simulink library "hgFilter"  (R2016b)
settings: Solver=VariableStepAuto  StartTime=0.0  StopTime=10.0  RelTol=1e-3
libraries: hgFilter x3
settings Model: Creator=Norris  LastModifiedBy=Norris

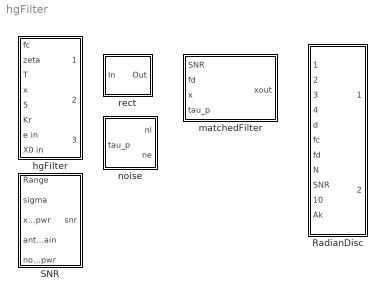
== system hgFilter ==
  RadianDisc : Subsystem
  SNR : Subsystem  Description=Calculates the SNR given several inputs, including range and RCS (sigma)
  hgFilter : Subsystem
  matchedFilter : Subsystem
  noise : Subsystem  Description=|
      | Takes in Tau_p and T (time step) and outputs all three noise coeffs. Note that currently Ak must be set 
      | in the workspace as 'Ak' for this block to function. Additionally, this version does not account for
      | multiple targets (there is only one Ak)
  rect : Subsystem  Description=Returns 1 if the mag of IN is 0.5 or less. Returns 0 otherwise

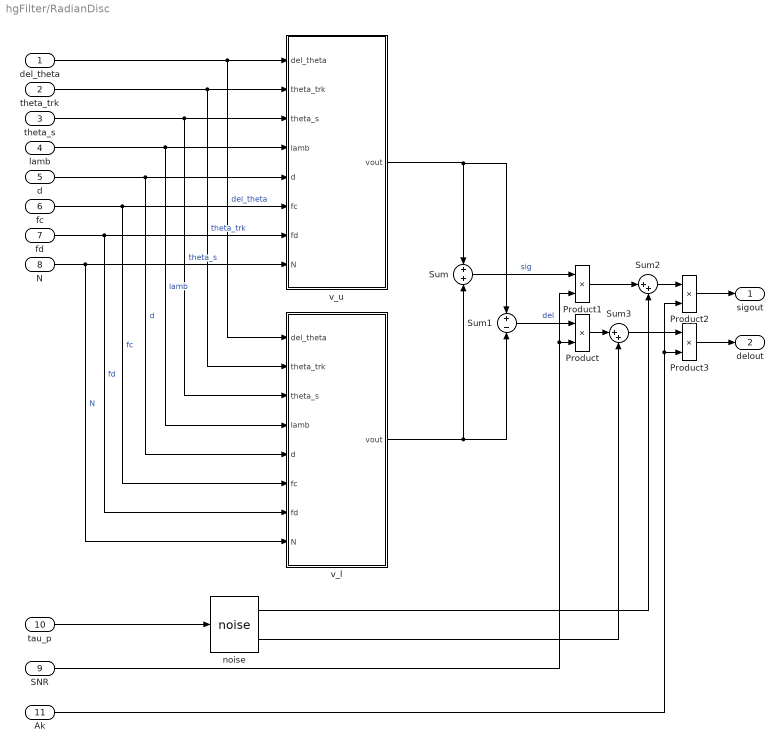
== system hgFilter/RadianDisc ==
  del_theta : Inport
  theta_trk : Inport  Port=2
  theta_s : Inport  Port=3
  lamb : Inport  Port=4
  d : Inport  Port=5
  fc : Inport  Port=6
  fd : Inport  Port=7
  N : Inport  Port=8
  SNR : Inport  Port=9
  tau_p : Inport  Port=10
  Ak : Inport  Port=11
  Product{,1..3} (4 alike) : Product
  Sum : Sum
  Sum1 : Sum  Inputs=+-
  Sum2 : Sum  Inputs=|++
  Sum3 : Sum  Inputs=|++
  noise : hgFilter/noise  Description=|
      | Takes in Tau_p and T (time step) and outputs all three noise coeffs. Note that currently Ak must be set 
      | in the workspace as 'Ak' for this block to function. Additionally, this version does not account for
      | multiple targets (there is only one Ak)
  v_l : Subsystem
  v_u : Subsystem
  sigout : Outport
  delout : Outport  Port=2
  wires:
  tau_p/1 -> noise/1
  Product2/1 -> sigout/1
  Sum3/1 -> Product3/1
  Sum2/1 -> Product2/1
  Product/1 -> Sum3/1
  Product1/1 -> Sum2/1
  del_theta/1 -> v_l/1(del_theta), v_u/1(del_theta)  "del_theta"
  theta_trk/1 -> v_l/2(theta_trk), v_u/2(theta_trk)  "theta_trk"
  theta_s/1 -> v_l/3(theta_s), v_u/3(theta_s)  "theta_s"
  lamb/1 -> v_l/4(lamb), v_u/4(lamb)  "lamb"
  d/1 -> v_l/5(d), v_u/5(d)  "d"
  fc/1 -> v_l/6(fc), v_u/6(fc)  "fc"
  fd/1 -> v_l/7(fd), v_u/7(fd)  "fd"
  N/1 -> v_l/8(N), v_u/8(N)  "N"
  v_l/1(vout) -> Sum1/2, Sum/2
  v_u/1(vout) -> Sum1/1, Sum/1
  Sum/1 -> Product1/1  "sig"
  Sum1/1 -> Product/1  "del"
  SNR/1 -> Product1/2, Product/2
  Product3/1 -> delout/1
  noise/1 -> Sum2/2
  noise/2 -> Sum3/2
  Ak/1 -> Product2/2, Product3/2

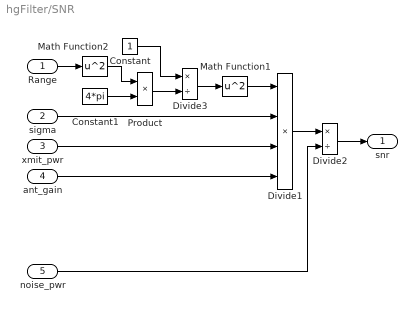
== system hgFilter/SNR ==
  Range : Inport
  sigma : Inport  Port=2
  xmit_pwr : Inport  Port=3
  ant_gain : Inport  Port=4
  noise_pwr : Inport  Port=5
  Constant : Constant
  Constant1 : Constant  Value=4*pi
  Divide1 : Product  Inputs=****
  Divide2 : Product  Inputs=*/
  Divide3 : Product  Inputs=*/
  Math Function1 : Math  Operator=square  SaturateOnIntegerOverflow=on
  Math Function2 : Math  Operator=square  SaturateOnIntegerOverflow=on
  Product : Product
  snr : Outport
  wires:
  Divide2/1 -> snr/1
  noise_pwr/1 -> Divide2/2
  xmit_pwr/1 -> Divide1/3
  sigma/1 -> Divide1/2
  ant_gain/1 -> Divide1/4
  Divide3/1 -> Math Function1/1
  Math Function1/1 -> Divide1/1
  Constant/1 -> Divide3/1
  Product/1 -> Divide3/2
  Range/1 -> Math Function2/1
  Constant1/1 -> Product/2
  Divide1/1 -> Divide2/1
  Math Function2/1 -> Product/1

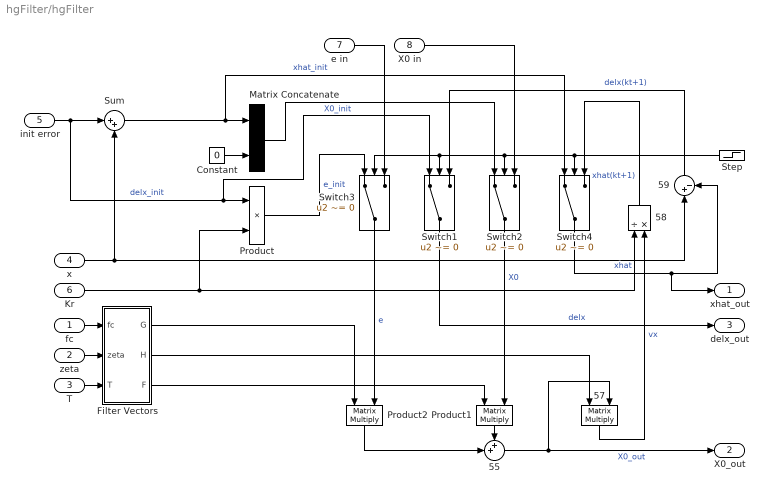
== system hgFilter/hgFilter ==
  fc : Inport
  zeta : Inport  Port=2
  T : Inport  Port=3
  x : Inport  Port=4
  init error : Inport  Port=5
  Kr : Inport  Port=6
  e in : Inport  Port=7
  X0 in : Inport  Port=8
  55 : Sum  Inputs=++|
  57 : Product  Multiplication=Matrix(*)
  58 : Product  Inputs=/*
  59 : Sum  Inputs=|+-
  Constant : Constant  Value=0
  Filter Vectors : Subsystem  TreatAsAtomicUnit=on
  Matrix Concatenate : Concatenate  Mode=Multidimensional array
  Product : Product
  Product1 : Product  Multiplication=Matrix(*)
  Product2 : Product  Multiplication=Matrix(*)
  Step : Step  Time=0.01  Before=1  After=0  SampleTime=0
  Sum : Sum  Inputs=|++
  Switch{1..4} (4 alike) : Switch  Criteria=u2 ~= 0  Threshold=0.5
  xhat_out : Outport
  X0_out : Outport  Port=2
  delx_out : Outport  Port=3
  wires:
  X0 in/1 -> Switch2/3
  59/1 -> Switch1/3  "delx(kt+1)"
  58/1 -> Switch4/3  "xhat(kt+1)"
  57/1 -> 58/2  "vx"
  Filter Vectors/2(H) -> 57/1
  55/1 -> 57/2, X0_out/1  "X0_out"
  Product2/1 -> 55/2
  Filter Vectors/1(G) -> Product2/1
  Product1/1 -> 55/1
  Filter Vectors/3(F) -> Product1/1
  e in/1 -> Switch3/3
  Switch4/1 -> xhat_out/1, 59/2  "xhat"
  Switch2/1 -> Product1/2  "X0"
  Switch3/1 -> Product2/2  "e"
  Step/1 -> Switch4/2, Switch3/2, Switch1/2, Switch2/2
  Product/1 -> Switch3/1  "e_init"
  Kr/1 -> 58/1, Product/2
  init error/1 -> Sum/1, Product/1, Switch1/1  "delx_init"
  x/1 -> Sum/2, 59/1
  Matrix Concatenate/1 -> Switch2/1  "X0_init"
  Constant/1 -> Matrix Concatenate/2
  Sum/1 -> Matrix Concatenate/1, Switch4/1  "xhat_init"
  fc/1 -> Filter Vectors/1(fc)
  zeta/1 -> Filter Vectors/2(zeta)
  T/1 -> Filter Vectors/3(T)
  Switch1/1 -> delx_out/1  "delx"

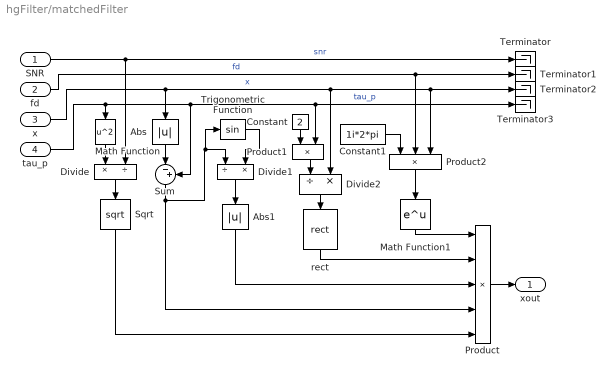
== system hgFilter/matchedFilter ==
  SNR : Inport
  fd : Inport  Port=2
  x : Inport  Port=3
  tau_p : Inport  Port=4
  Abs : Abs
  Abs1 : Abs
  Constant : Constant  Value=2
  Constant1 : Constant  Value=1i*2*pi
  Divide : Product  Inputs=*/
  Divide1 : Product  Inputs=/*
  Divide2 : Product  Inputs=/*
  Math Function : Math  Operator=square  SaturateOnIntegerOverflow=on
  Math Function1 : Math  SaturateOnIntegerOverflow=on
  Product : Product  Inputs=5
  Product1 : Product
  Product2 : Product  Inputs=3
  Sqrt : Sqrt  SaturateOnIntegerOverflow=on
  Sum : Sum  Inputs=|-+
  Terminator{,1..3} (4 alike) : Terminator
  Trigonometric Function : Trigonometry
  rect : hgFilter/rect
  xout : Outport
  wires:
  SNR/1 -> Terminator/1, Divide/2  "snr"
  fd/1 -> Terminator1/1, Product2/2  "fd"
  x/1 -> Abs/1, Terminator2/1, Product2/3, Divide2/2  "x"
  tau_p/1 -> Math Function/1, Sum/2, Product1/2, Terminator3/1  "tau_p"
  Math Function/1 -> Divide/1
  Divide/1 -> Sqrt/1
  Abs/1 -> Sum/1
  Sqrt/1 -> Product/5
  Sum/1 -> Divide1/1, Trigonometric Function/1, Product/4
  Trigonometric Function/1 -> Divide1/2
  Divide1/1 -> Abs1/1
  Abs1/1 -> Product/3
  Constant/1 -> Product1/1
  Product1/1 -> Divide2/1
  Divide2/1 -> rect/1
  rect/1 -> Product/2
  Constant1/1 -> Product2/1
  Product2/1 -> Math Function1/1
  Math Function1/1 -> Product/1
  Product/1 -> xout/1

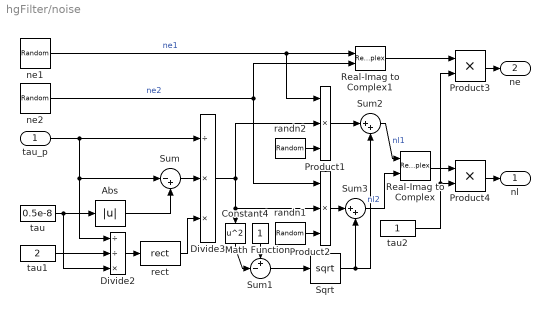
== system hgFilter/noise ==
  tau_p : Inport
  Abs : Abs
  Constant4 : Constant
  Divide2 : Product  Inputs=//*
  Divide3 : Product  Inputs=/**
  Math Function : Math  Operator=square  SaturateOnIntegerOverflow=on
  Product1 : Product  Inputs=3
  Product2 : Product  Inputs=3
  Product3 : Product
  Product4 : Product
  Real-Imag to Complex : RealImagToComplex
  Real-Imag to Complex1 : RealImagToComplex
  Sqrt : Sqrt  SaturateOnIntegerOverflow=on
  Sum : Sum  Inputs=|-+
  Sum1 : Sum  Inputs=+-|
  Sum2 : Sum  Inputs=|++
  Sum3 : Sum  Inputs=|++
  ne1 : RandomNumber  SampleTime=0.1
  ne2 : RandomNumber  SampleTime=0.1
  randn1 : RandomNumber  SampleTime=0.1
  randn2 : RandomNumber  SampleTime=0.1
  rect : hgFilter/rect  Description=Returns 1 if the mag of IN is 0.5 or less. Returns 0 otherwise
  tau : Constant  Value=0.5e-8
  tau1 : Constant  Value=2
  tau2 : Constant
  nl : Outport
  ne : Outport  Port=2
  wires:
  tau/1 -> Divide2/3, Abs/1
  Abs/1 -> Sum/2
  Sum/1 -> Divide3/2
  tau_p/1 -> Divide3/1, Divide2/1, Sum/1
  rect/1 -> Divide3/3
  tau1/1 -> Divide2/2
  Divide2/1 -> rect/1
  ne1/1 -> Real-Imag to Complex1/1, Product1/1  "ne1"
  ne2/1 -> Real-Imag to Complex1/2, Product2/1  "ne2"
  Divide3/1 -> Product2/2, Math Function/1, Product1/2
  randn2/1 -> Product1/3
  randn1/1 -> Product2/3
  Math Function/1 -> Sum1/2
  Constant4/1 -> Sum1/1
  Sum1/1 -> Sqrt/1
  Product1/1 -> Sum2/1
  Product2/1 -> Sum3/1
  Sqrt/1 -> Sum3/2, Sum2/2
  Sum2/1 -> Real-Imag to Complex/1  "nl1"
  Sum3/1 -> Real-Imag to Complex/2  "nl2"
  Real-Imag to Complex1/1 -> Product3/1
  Real-Imag to Complex/1 -> Product4/1
  Product4/1 -> nl/1
  Product3/1 -> ne/1
  tau2/1 -> Product3/2, Product4/2

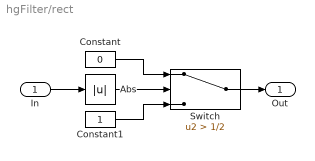
== system hgFilter/rect ==
  In : Inport
  Abs : Abs
  Constant : Constant  Value=0
  Constant1 : Constant
  Switch : Switch  Criteria=u2 > Threshold  Threshold=1/2
  Out : Outport
  wires:
  In/1 -> Abs/1
  Abs/1 -> Switch/2
  Constant1/1 -> Switch/3
  Constant/1 -> Switch/1
  Switch/1 -> Out/1

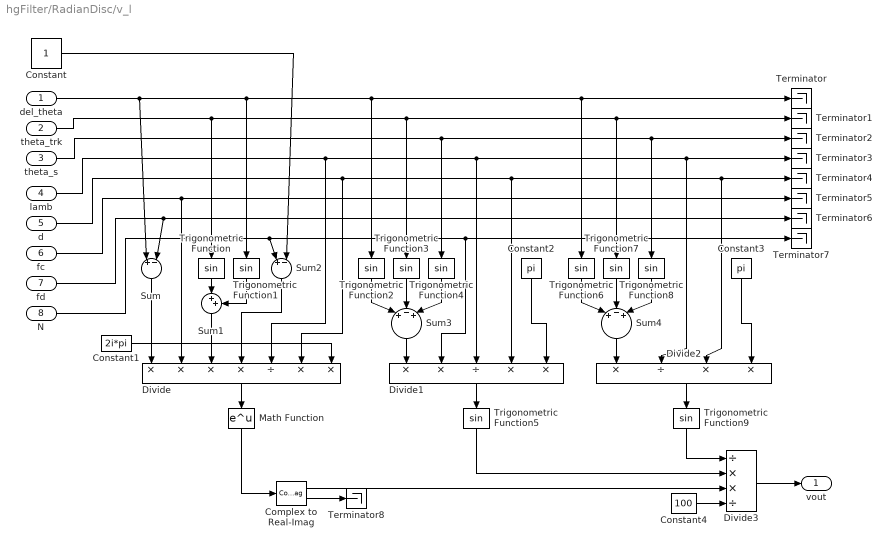
== system hgFilter/RadianDisc/v_l ==
  del_theta : Inport
  theta_trk : Inport  Port=2
  theta_s : Inport  Port=3
  lamb : Inport  Port=4
  d : Inport  Port=5
  fc : Inport  Port=6
  fd : Inport  Port=7
  N : Inport  Port=8
  Complex to Real-Imag : ComplexToRealImag
  Constant : Constant
  Constant1 : Constant  Value=2i*pi
  Constant2 : Constant  Value=pi
  Constant3 : Constant  Value=pi
  Constant4 : Constant  Value=100
  Divide : Product  Inputs=****/**
  Divide1 : Product  Inputs=**/**
  Divide2 : Product  Inputs=*/**
  Divide3 : Product  Inputs=/**/
  Math Function : Math  SaturateOnIntegerOverflow=on
  Sum : Sum  Inputs=|+-|
  Sum1 : Sum  Inputs=|++
  Sum2 : Sum  Inputs=|+-|
  Sum3 : Sum  Inputs=|+-+|
  Sum4 : Sum  Inputs=|+-+|
  Terminator{,1..8} (9 alike) : Terminator
  Trigonometric Function{,1..9} (10 alike) : Trigonometry
  vout : Outport
  wires:
  Constant4/1 -> Divide3/4
  Sum4/1 -> Divide2/1
  Sum2/1 -> Divide/4
  fd/1 -> Terminator6/1, Sum/2
  Trigonometric Function2/1 -> Sum3/1
  Trigonometric Function7/1 -> Sum4/2
  del_theta/1 -> Trigonometric Function2/1, Trigonometric Function6/1, Terminator/1, Trigonometric Function1/1, Sum/1
  Divide2/1 -> Trigonometric Function9/1
  d/1 -> Divide1/4, Divide2/3, Terminator4/1, Divide/6
  fc/1 -> Terminator5/1, Divide/2
  Sum/1 -> Divide/1
  Divide/1 -> Math Function/1
  Trigonometric Function8/1 -> Sum4/3
  Divide1/1 -> Trigonometric Function5/1
  Trigonometric Function9/1 -> Divide3/1
  theta_trk/1 -> Trigonometric Function3/1, Terminator1/1, Trigonometric Function7/1, Trigonometric Function/1
  N/1 -> Divide1/2, Terminator7/1, Sum2/1
  Trigonometric Function1/1 -> Sum1/2
  Constant/1 -> Sum2/2
  Sum1/1 -> Divide/3
  lamb/1 -> Divide/5, Divide2/2, Terminator3/1, Divide1/3
  Constant1/1 -> Divide/7
  Trigonometric Function5/1 -> Divide3/2
  Trigonometric Function6/1 -> Sum4/1
  Divide3/1 -> vout/1
  theta_s/1 -> Trigonometric Function8/1, Terminator2/1, Trigonometric Function4/1
  Trigonometric Function4/1 -> Sum3/3
  Trigonometric Function3/1 -> Sum3/2
  Sum3/1 -> Divide1/1
  Constant2/1 -> Divide1/5
  Constant3/1 -> Divide2/4
  Trigonometric Function/1 -> Sum1/1
  Complex to Real-Imag/1 -> Divide3/3
  Math Function/1 -> Complex to Real-Imag/1
  Complex to Real-Imag/2 -> Terminator8/1

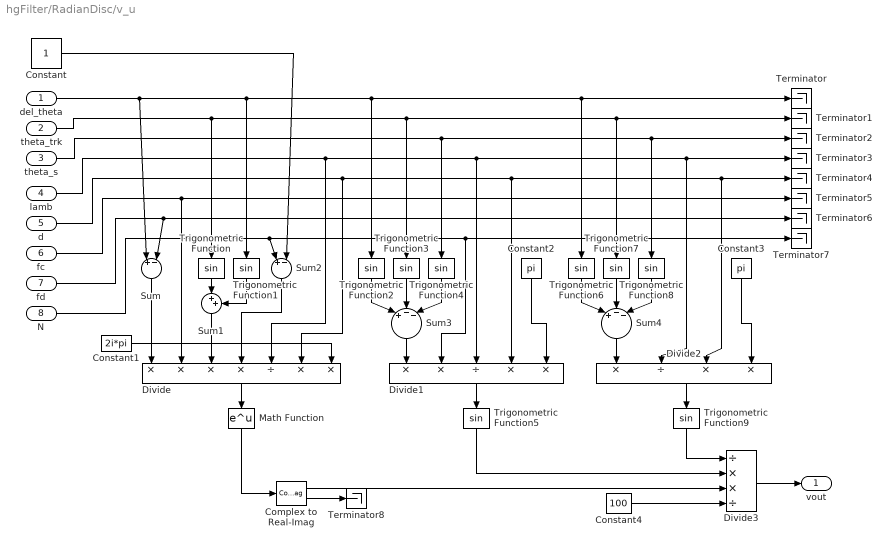
== system hgFilter/RadianDisc/v_u ==
  del_theta : Inport
  theta_trk : Inport  Port=2
  theta_s : Inport  Port=3
  lamb : Inport  Port=4
  d : Inport  Port=5
  fc : Inport  Port=6
  fd : Inport  Port=7
  N : Inport  Port=8
  Complex to Real-Imag : ComplexToRealImag
  Constant : Constant
  Constant1 : Constant  Value=2i*pi
  Constant2 : Constant  Value=pi
  Constant3 : Constant  Value=pi
  Constant4 : Constant  Value=100
  Divide : Product  Inputs=****/**
  Divide1 : Product  Inputs=**/**
  Divide2 : Product  Inputs=*/**
  Divide3 : Product  Inputs=/**/
  Math Function : Math  SaturateOnIntegerOverflow=on
  Sum : Sum  Inputs=|+-|
  Sum1 : Sum  Inputs=|++
  Sum2 : Sum  Inputs=|+-|
  Sum3 : Sum  Inputs=|+--|
  Sum4 : Sum  Inputs=|+--|
  Terminator{,1..8} (9 alike) : Terminator
  Trigonometric Function{,1..9} (10 alike) : Trigonometry
  vout : Outport
  wires:
  Constant4/1 -> Divide3/4
  Sum4/1 -> Divide2/1
  Sum2/1 -> Divide/4
  fd/1 -> Terminator6/1, Sum/2
  Trigonometric Function2/1 -> Sum3/1
  Trigonometric Function7/1 -> Sum4/2
  del_theta/1 -> Trigonometric Function2/1, Trigonometric Function6/1, Terminator/1, Trigonometric Function1/1, Sum/1
  Divide2/1 -> Trigonometric Function9/1
  d/1 -> Divide1/4, Divide2/3, Terminator4/1, Divide/6
  fc/1 -> Terminator5/1, Divide/2
  Sum/1 -> Divide/1
  Divide/1 -> Math Function/1
  Trigonometric Function8/1 -> Sum4/3
  Divide1/1 -> Trigonometric Function5/1
  Trigonometric Function9/1 -> Divide3/1
  theta_trk/1 -> Trigonometric Function3/1, Terminator1/1, Trigonometric Function7/1, Trigonometric Function/1
  N/1 -> Divide1/2, Terminator7/1, Sum2/1
  Trigonometric Function1/1 -> Sum1/2
  Constant/1 -> Sum2/2
  Sum1/1 -> Divide/3
  Complex to Real-Imag/1 -> Divide3/3
  lamb/1 -> Divide/5, Divide2/2, Terminator3/1, Divide1/3
  Constant1/1 -> Divide/7
  Trigonometric Function5/1 -> Divide3/2
  Trigonometric Function6/1 -> Sum4/1
  Divide3/1 -> vout/1
  theta_s/1 -> Trigonometric Function8/1, Terminator2/1, Trigonometric Function4/1
  Trigonometric Function4/1 -> Sum3/3
  Trigonometric Function3/1 -> Sum3/2
  Sum3/1 -> Divide1/1
  Constant2/1 -> Divide1/5
  Constant3/1 -> Divide2/4
  Trigonometric Function/1 -> Sum1/1
  Math Function/1 -> Complex to Real-Imag/1
  Complex to Real-Imag/2 -> Terminator8/1

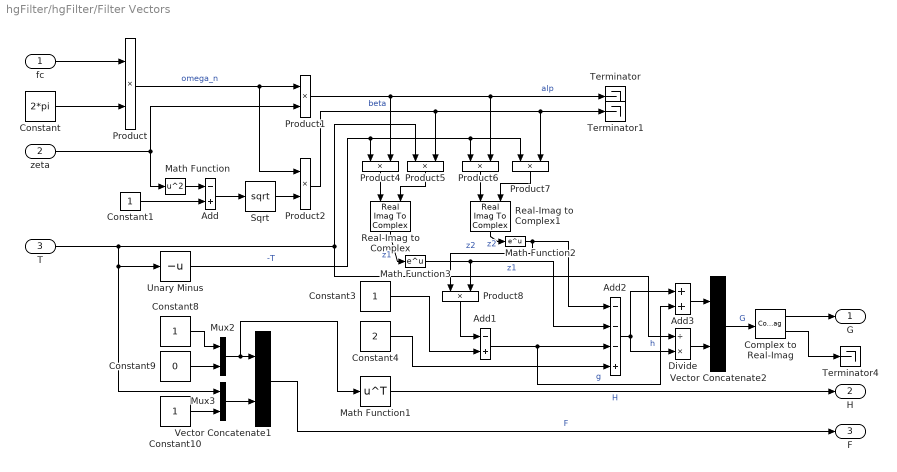
== system hgFilter/hgFilter/Filter Vectors ==
  fc : Inport
  zeta : Inport  Port=2
  T : Inport  Port=3
  Add : Sum  Inputs=-+
  Add1 : Sum  Inputs=-+
  Add2 : Sum  Inputs=---+
  Add3 : Sum
  Complex to Real-Imag : ComplexToRealImag
  Constant : Constant  Value=2*pi
  Constant{1,3,8,10} (4 alike) : Constant
  Constant4 : Constant  Value=2
  Constant9 : Constant  Value=0
  Divide : Product  Inputs=/*
  Math Function : Math  Operator=square  SaturateOnIntegerOverflow=on
  Math Function1 : Math  Operator=transpose  SaturateOnIntegerOverflow=on
  Math Function2 : Math  OutputSignalType=complex  SaturateOnIntegerOverflow=on
  Math Function3 : Math  OutputSignalType=complex  SaturateOnIntegerOverflow=on
  Mux2 : Mux  Inputs=2
  Mux3 : Mux  Inputs=2
  Product{,1..2,4..8} (8 alike) : Product
  Real-Imag to Complex : RealImagToComplex
  Real-Imag to Complex1 : RealImagToComplex
  Sqrt : Sqrt  SaturateOnIntegerOverflow=on
  Terminator : Terminator
  Terminator1 : Terminator
  Terminator4 : Terminator
  Unary Minus : UnaryMinus
  Vector Concatenate1 : Concatenate  Mode=Multidimensional array  ConcatenateDimension=2
  Vector Concatenate2 : Concatenate  Mode=Multidimensional array
  G : Outport
  H : Outport  Port=2
  F : Outport  Port=3
  wires:
  Complex to Real-Imag/2 -> Terminator4/1
  Complex to Real-Imag/1 -> G/1
  Real-Imag to Complex1/1 -> Math Function2/1  "z2"
  Math Function3/1 -> Add2/2, Product8/2  "z1"
  Product7/1 -> Real-Imag to Complex1/2
  Divide/1 -> Vector Concatenate2/2
  Unary Minus/1 -> Product7/1, Product6/1, Product4/1  "-T"
  Product/1 -> Product2/1, Product1/1  "omega_n"
  Add3/1 -> Vector Concatenate2/1
  Product4/1 -> Real-Imag to Complex/1
  Constant1/1 -> Add/2
  Product8/1 -> Add1/1
  zeta/1 -> Math Function/1, Product1/2
  Constant9/1 -> Mux2/2
  Math Function/1 -> Add/1
  Vector Concatenate1/1 -> F/1  "F"
  Product1/1 -> Terminator/1, Product6/2, Product4/2  "alp"
  Constant4/1 -> Add2/4
  Product2/1 -> Terminator1/1, Product7/2, Product5/2  "beta"
  Constant/1 -> Product/2
  fc/1 -> Product/1
  Product5/1 -> Real-Imag to Complex/2
  Constant8/1 -> Mux2/1
  Add/1 -> Sqrt/1
  Product6/1 -> Real-Imag to Complex1/1
  Constant3/1 -> Add1/2
  Add2/1 -> Divide/2, Add3/1  "h"
  Mux3/1 -> Vector Concatenate1/2
  Math Function2/1 -> Product8/1, Add2/1  "z2"
  Real-Imag to Complex/1 -> Math Function3/1  "z1"
  Add1/1 -> Add3/2, Add2/3  "g"
  Mux2/1 -> Math Function1/1, Vector Concatenate1/1
  Constant10/1 -> Mux3/2
  T/1 -> Product5/1, Divide/1, Mux3/1, Unary Minus/1
  Sqrt/1 -> Product2/2
  Math Function1/1 -> H/1  "H"
  Vector Concatenate2/1 -> Complex to Real-Imag/1  "G"
